simulink model "stereo_ibvs_core_before_04_kinematics_20260723_212009"  (R2025b)
settings: Solver=FixedStepDiscrete  StartTime=0.0  StopTime=inf  FixedStep=cfg.Ts  RelTol=1e-3
InitFcn:
  | cfgValid__=evalin('base','exist(''cfg'',''var'')==1 && isstruct(cfg) && all(isfield(cfg,{''Ts'',''robot'',''qInitial'',''zoomInitialSteps'',''cameraIntrinsicsStage1'',''rhoD'',''stereoBaseline'',''centerDesired'',''Kc'',''lambdaC'',''qMin'',''qMax'',''qLimitSoftMargin'',''qDotAlgorithmMax'',''stage1CalibrationReady''}))');if ~cfgValid__,modelFile__=get_param(bdroot,'FileName');modelDir__=fileparts(modelFile__);config1__=fullfile(modelDir__,'stereo_ibvs_config.m');config2__=fullfile(fileparts(modelDir__),'config','stereo_ibvs_config.m');if isfile(config1__),run(config1__);elseif isfile(config2__),run(config2__);else,error('StereoIBVS:ConfigNotFound','找不到stereo_ibvs_config.m。');end;end;clear cfgValid__ modelFile__ modelDir__ config1__ config2__
undefined symbols (not defined in the file): cfg
(part 1 of 2)
settings Model: Creator=harry  LastModifiedBy=harry

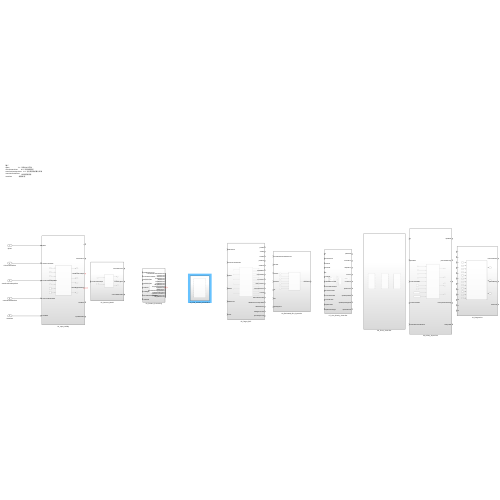
[thumbnail: Simulink's stored preview of the top-level diagram]
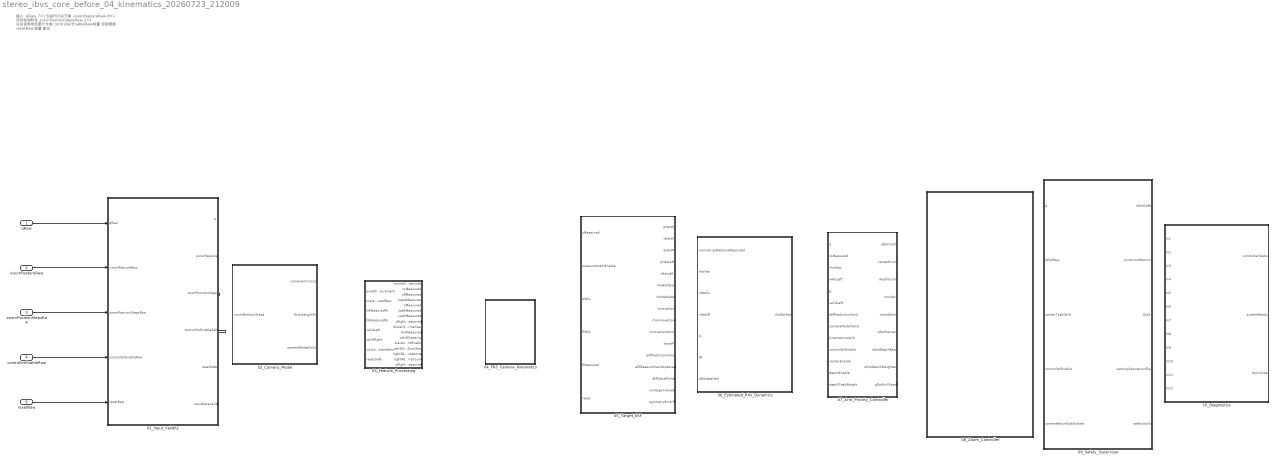
== system stereo_ibvs_core_before_04_kinematics_20260723_212009 ==
  note: 输入:
      | qRaw 7×1 当前FR3关节角
      | visionFeatureRaw 8×1 双目检测特征
      | zoomPositionStepsRaw 2×1 左右变焦电机累计步数
      | controllerEnableRaw 标量 控制使能
      | resetRaw 标量 复位
  qRaw : Inport  OutDataTypeStr=double  PortDimensions=[7 1]
  visionFeatureRaw : Inport  Port=2  PortDimensions=[8 1]
  zoomPositionStepsRaw : Inport  Port=3  PortDimensions=[2 1]
  controllerEnableRaw : Inport  Port=4  OutDataTypeStr=double  PortDimensions=1
  resetRaw : Inport  Port=5  OutDataTypeStr=double  PortDimensions=1
  01_Input_Validity : Subsystem
  02_Camera_Model : Subsystem
  03_Feature_Processing : Subsystem  Description=将像素坐标转换为左右相机归一化坐标，并检查输入有效性。
  04_FR3_Camera_Kinematics : Subsystem
  05_Target_EKF : Subsystem
  06_Estimated_Rho_Dynamics : Subsystem
  07_Arm_Priority_Controller : Subsystem
  08_Zoom_Controller : Subsystem
  09_Safety_Supervisor : Subsystem
  10_Diagnostics : Subsystem
  wires:
  resetRaw/1 -> 01_Input_Validity/5(resetRaw)
  controllerEnableRaw/1 -> 01_Input_Validity/4(controllerEnableRaw)
  zoomPositionStepsRaw/1 -> 01_Input_Validity/3(zoomPositionStepsRaw)
  visionFeatureRaw/1 -> 01_Input_Validity/2(visionFeatureRaw)
  01_Input_Validity/4(controllerEnableSafe) -> ?
  qRaw/1 -> 01_Input_Validity/1(qRaw)
  ? -> ?
  01_Input_Validity/3(zoomPositionSteps) -> ?

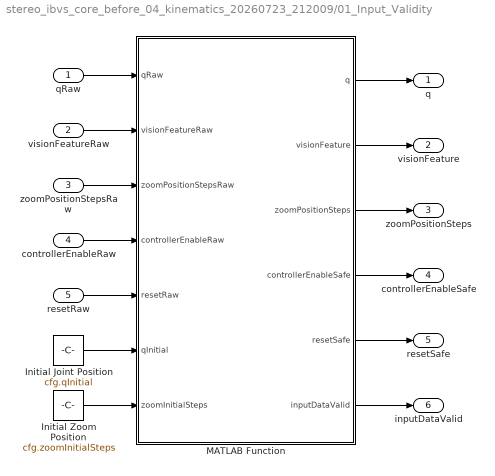
== system stereo_ibvs_core_before_04_kinematics_20260723_212009/01_Input_Validity ==
  qRaw : Inport  PortDimensions=[7 1]
  visionFeatureRaw : Inport  Port=2  PortDimensions=[8 1]
  zoomPositionStepsRaw : Inport  Port=3  PortDimensions=[2 1]
  controllerEnableRaw : Inport  Port=4  PortDimensions=1
  resetRaw : Inport  Port=5  PortDimensions=1
  Initial Joint Position : Constant  Value=cfg.qInitial  VectorParams1D=off
  Initial Zoom Position : Constant  Value=cfg.zoomInitialSteps  VectorParams1D=off
  MATLAB Function : MATLAB Function  TreatAsAtomicUnit=on
  q : Outport  PortDimensions=[7 1]
  visionFeature : Outport  Port=2  PortDimensions=[8 1]
  zoomPositionSteps : Outport  Port=3  PortDimensions=[2 1]
  controllerEnableSafe : Outport  Port=4  PortDimensions=1
  resetSafe : Outport  Port=5  PortDimensions=1
  inputDataValid : Outport  Port=6  PortDimensions=1
  wires:
  MATLAB Function/1(q) -> q/1
  MATLAB Function/2(visionFeature) -> visionFeature/1
  MATLAB Function/3(zoomPositionSteps) -> zoomPositionSteps/1
  MATLAB Function/4(controllerEnableSafe) -> controllerEnableSafe/1
  MATLAB Function/5(resetSafe) -> resetSafe/1
  MATLAB Function/6(inputDataValid) -> inputDataValid/1
  qRaw/1 -> MATLAB Function/1(qRaw)
  visionFeatureRaw/1 -> MATLAB Function/2(visionFeatureRaw)
  zoomPositionStepsRaw/1 -> MATLAB Function/3(zoomPositionStepsRaw)
  controllerEnableRaw/1 -> MATLAB Function/4(controllerEnableRaw)
  resetRaw/1 -> MATLAB Function/5(resetRaw)
  Initial Joint Position/1 -> MATLAB Function/6(qInitial)
  Initial Zoom Position/1 -> MATLAB Function/7(zoomInitialSteps)

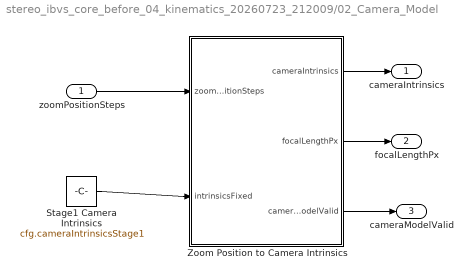
== system stereo_ibvs_core_before_04_kinematics_20260723_212009/02_Camera_Model ==
  zoomPositionSteps : Inport  PortDimensions=[2 1]
  Stage1 Camera Intrinsics : Constant  Value=cfg.cameraIntrinsicsStage1  VectorParams1D=off
  Zoom Position to Camera Intrinsics : MATLAB Function  TreatAsAtomicUnit=on
  cameraIntrinsics : Outport  PortDimensions=[8 1]
  focalLengthPx : Outport  Port=2  PortDimensions=[2 1]
  cameraModelValid : Outport  Port=3  PortDimensions=1
  wires:
  zoomPositionSteps/1 -> Zoom Position to Camera Intrinsics/1(zoomPositionSteps)
  Stage1 Camera Intrinsics/1 -> Zoom Position to Camera Intrinsics/2(intrinsicsFixed)
  Zoom Position to Camera Intrinsics/3(cameraModelValid) -> cameraModelValid/1
  Zoom Position to Camera Intrinsics/2(focalLengthPx) -> focalLengthPx/1
  Zoom Position to Camera Intrinsics/1(cameraIntrinsics) -> cameraIntrinsics/1

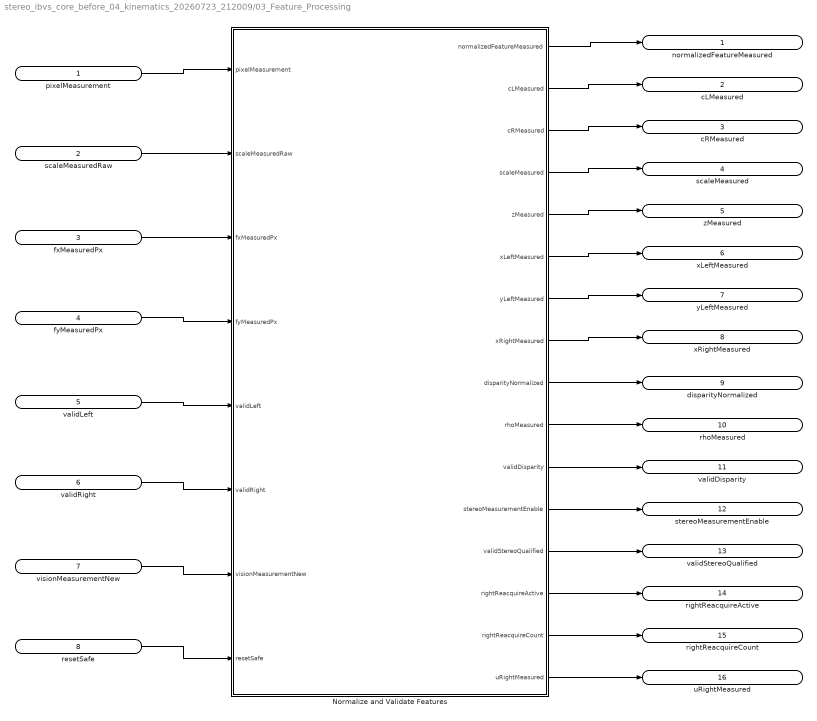
== system stereo_ibvs_core_before_04_kinematics_20260723_212009/03_Feature_Processing ==
  pixelMeasurement : Inport  OutDataTypeStr=double  PortDimensions=[4 1]
  scaleMeasuredRaw : Inport  Port=2  OutDataTypeStr=double  PortDimensions=[2 1]
  fxMeasuredPx : Inport  Port=3  OutDataTypeStr=double  PortDimensions=[2 1]
  fyMeasuredPx : Inport  Port=4  OutDataTypeStr=double  PortDimensions=[2 1]
  validLeft : Inport  Port=5  OutDataTypeStr=double  PortDimensions=[1 1]
  validRight : Inport  Port=6  OutDataTypeStr=double  PortDimensions=[1 1]
  visionMeasurementNew : Inport  Port=7  OutDataTypeStr=double  PortDimensions=[1 1]
  resetSafe : Inport  Port=8  OutDataTypeStr=double  PortDimensions=[1 1]
  Normalize and Validate Features : MATLAB Function  TreatAsAtomicUnit=on
  normalizedFeatureMeasured : Outport  PortDimensions=[4 1]
  cLMeasured : Outport  Port=2  PortDimensions=[2 1]
  cRMeasured : Outport  Port=3  PortDimensions=[2 1]
  scaleMeasured : Outport  Port=4  PortDimensions=[2 1]
  zMeasured : Outport  Port=5  PortDimensions=[3 1]
  xLeftMeasured : Outport  Port=6  PortDimensions=[1 1]
  yLeftMeasured : Outport  Port=7  PortDimensions=[1 1]
  xRightMeasured : Outport  Port=8  PortDimensions=[1 1]
  disparityNormalized : Outport  Port=9  PortDimensions=[1 1]
  rhoMeasured : Outport  Port=10  PortDimensions=[1 1]
  validDisparity : Outport  Port=11  PortDimensions=[1 1]
  stereoMeasurementEnable : Outport  Port=12  PortDimensions=[1 1]
  validStereoQualified : Outport  Port=13  PortDimensions=[1 1]
  rightReacquireActive : Outport  Port=14  PortDimensions=[1 1]
  rightReacquireCount : Outport  Port=15  PortDimensions=[1 1]
  uRightMeasured : Outport  Port=16  PortDimensions=[1 1]
  wires:
  pixelMeasurement/1 -> Normalize and Validate Features/1(pixelMeasurement)
  scaleMeasuredRaw/1 -> Normalize and Validate Features/2(scaleMeasuredRaw)
  fxMeasuredPx/1 -> Normalize and Validate Features/3(fxMeasuredPx)
  fyMeasuredPx/1 -> Normalize and Validate Features/4(fyMeasuredPx)
  validLeft/1 -> Normalize and Validate Features/5(validLeft)
  validRight/1 -> Normalize and Validate Features/6(validRight)
  visionMeasurementNew/1 -> Normalize and Validate Features/7(visionMeasurementNew)
  resetSafe/1 -> Normalize and Validate Features/8(resetSafe)
  Normalize and Validate Features/2(cLMeasured) -> cLMeasured/1
  Normalize and Validate Features/3(cRMeasured) -> cRMeasured/1
  Normalize and Validate Features/4(scaleMeasured) -> scaleMeasured/1
  Normalize and Validate Features/5(zMeasured) -> zMeasured/1
  Normalize and Validate Features/6(xLeftMeasured) -> xLeftMeasured/1
  Normalize and Validate Features/7(yLeftMeasured) -> yLeftMeasured/1
  Normalize and Validate Features/8(xRightMeasured) -> xRightMeasured/1
  Normalize and Validate Features/9(disparityNormalized) -> disparityNormalized/1
  Normalize and Validate Features/10(rhoMeasured) -> rhoMeasured/1
  Normalize and Validate Features/11(validDisparity) -> validDisparity/1
  Normalize and Validate Features/12(stereoMeasurementEnable) -> stereoMeasurementEnable/1
  Normalize and Validate Features/13(validStereoQualified) -> validStereoQualified/1
  Normalize and Validate Features/14(rightReacquireActive) -> rightReacquireActive/1
  Normalize and Validate Features/15(rightReacquireCount) -> rightReacquireCount/1
  Normalize and Validate Features/16(uRightMeasured) -> uRightMeasured/1
  Normalize and Validate Features/1(normalizedFeatureMeasured) -> normalizedFeatureMeasured/1

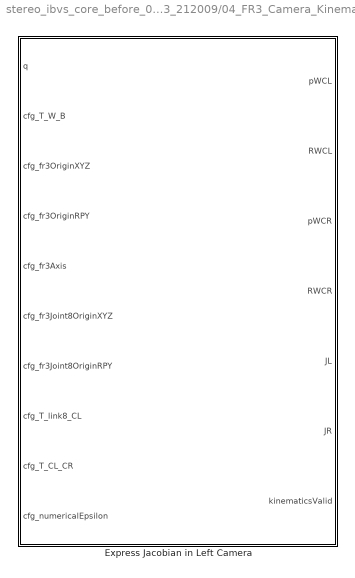
== system stereo_ibvs_core_before_04_kinematics_20260723_212009/04_FR3_Camera_Kinematics ==
  Express Jacobian in Left Camera : MATLAB Function  TreatAsAtomicUnit=on

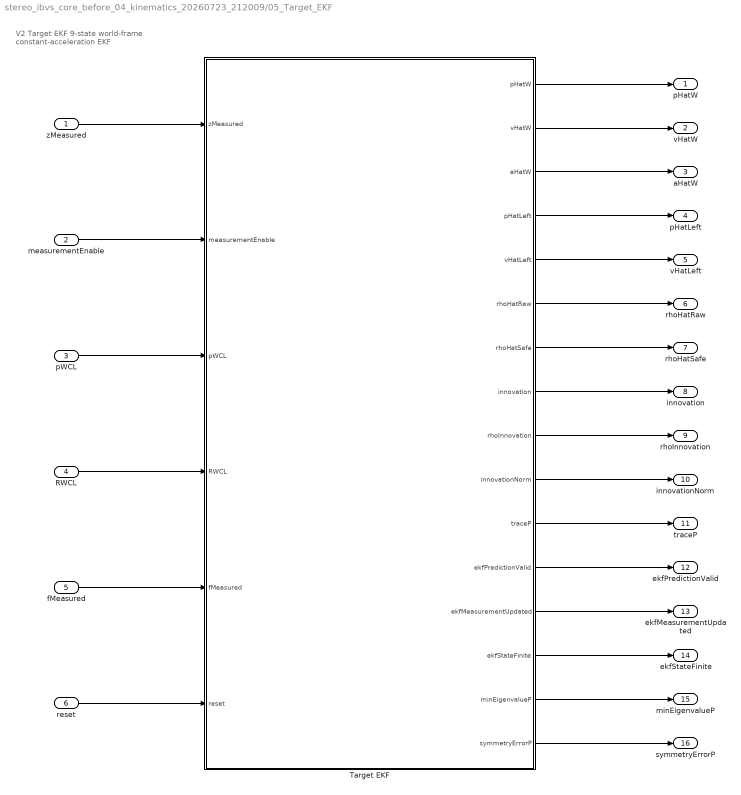
== system stereo_ibvs_core_before_04_kinematics_20260723_212009/05_Target_EKF ==
  note: V2 Target EKF
      | 9-state world-frame constant-acceleration EKF
  zMeasured : Inport  OutDataTypeStr=double  PortDimensions=3
  measurementEnable : Inport  Port=2  OutDataTypeStr=double  PortDimensions=1
  pWCL : Inport  Port=3  OutDataTypeStr=double  PortDimensions=3
  RWCL : Inport  Port=4  OutDataTypeStr=double  PortDimensions=[3 3]
  fMeasured : Inport  Port=5  OutDataTypeStr=double  PortDimensions=2
  reset : Inport  Port=6  OutDataTypeStr=double  PortDimensions=1
  Target EKF : MATLAB Function  TreatAsAtomicUnit=on
  pHatW : Outport
  vHatW : Outport  Port=2
  aHatW : Outport  Port=3
  pHatLeft : Outport  Port=4
  vHatLeft : Outport  Port=5
  rhoHatRaw : Outport  Port=6
  rhoHatSafe : Outport  Port=7
  innovation : Outport  Port=8
  rhoInnovation : Outport  Port=9
  innovationNorm : Outport  Port=10
  traceP : Outport  Port=11
  ekfPredictionValid : Outport  Port=12
  ekfMeasurementUpdated : Outport  Port=13
  ekfStateFinite : Outport  Port=14
  minEigenvalueP : Outport  Port=15
  symmetryErrorP : Outport  Port=16
  wires:
  zMeasured/1 -> Target EKF/1(zMeasured)
  measurementEnable/1 -> Target EKF/2(measurementEnable)
  pWCL/1 -> Target EKF/3(pWCL)
  RWCL/1 -> Target EKF/4(RWCL)
  fMeasured/1 -> Target EKF/5(fMeasured)
  reset/1 -> Target EKF/6(reset)
  Target EKF/1(pHatW) -> pHatW/1
  Target EKF/2(vHatW) -> vHatW/1
  Target EKF/3(aHatW) -> aHatW/1
  Target EKF/4(pHatLeft) -> pHatLeft/1
  Target EKF/5(vHatLeft) -> vHatLeft/1
  Target EKF/6(rhoHatRaw) -> rhoHatRaw/1
  Target EKF/7(rhoHatSafe) -> rhoHatSafe/1
  Target EKF/8(innovation) -> innovation/1
  Target EKF/9(rhoInnovation) -> rhoInnovation/1
  Target EKF/10(innovationNorm) -> innovationNorm/1
  Target EKF/11(traceP) -> traceP/1
  Target EKF/12(ekfPredictionValid) -> ekfPredictionValid/1
  Target EKF/13(ekfMeasurementUpdated) -> ekfMeasurementUpdated/1
  Target EKF/14(ekfStateFinite) -> ekfStateFinite/1
  Target EKF/15(minEigenvalueP) -> minEigenvalueP/1
  Target EKF/16(symmetryErrorP) -> symmetryErrorP/1

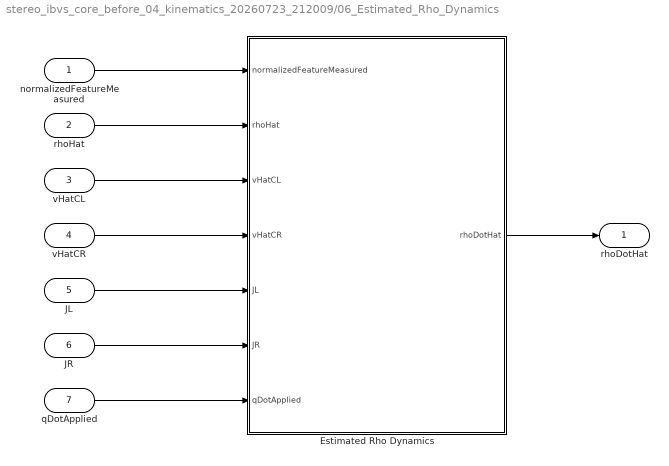
== system stereo_ibvs_core_before_04_kinematics_20260723_212009/06_Estimated_Rho_Dynamics ==
  normalizedFeatureMeasured : Inport  OutDataTypeStr=double  PortDimensions=[4 1]
  rhoHat : Inport  Port=2  OutDataTypeStr=double  PortDimensions=1
  vHatCL : Inport  Port=3  OutDataTypeStr=double  PortDimensions=[3 1]
  vHatCR : Inport  Port=4  OutDataTypeStr=double  PortDimensions=[3 1]
  JL : Inport  Port=5  OutDataTypeStr=double  PortDimensions=[6 7]
  JR : Inport  Port=6  OutDataTypeStr=double  PortDimensions=[6 7]
  qDotApplied : Inport  Port=7  OutDataTypeStr=double  PortDimensions=[7 1]
  Estimated Rho Dynamics : MATLAB Function  TreatAsAtomicUnit=on
  rhoDotHat : Outport  OutDataTypeStr=double  PortDimensions=[2 1]
  wires:
  normalizedFeatureMeasured/1 -> Estimated Rho Dynamics/1(normalizedFeatureMeasured)
  rhoHat/1 -> Estimated Rho Dynamics/2(rhoHat)
  vHatCL/1 -> Estimated Rho Dynamics/3(vHatCL)
  vHatCR/1 -> Estimated Rho Dynamics/4(vHatCR)
  JL/1 -> Estimated Rho Dynamics/5(JL)
  JR/1 -> Estimated Rho Dynamics/6(JR)
  qDotApplied/1 -> Estimated Rho Dynamics/7(qDotApplied)
  Estimated Rho Dynamics/1(rhoDotHat) -> rhoDotHat/1

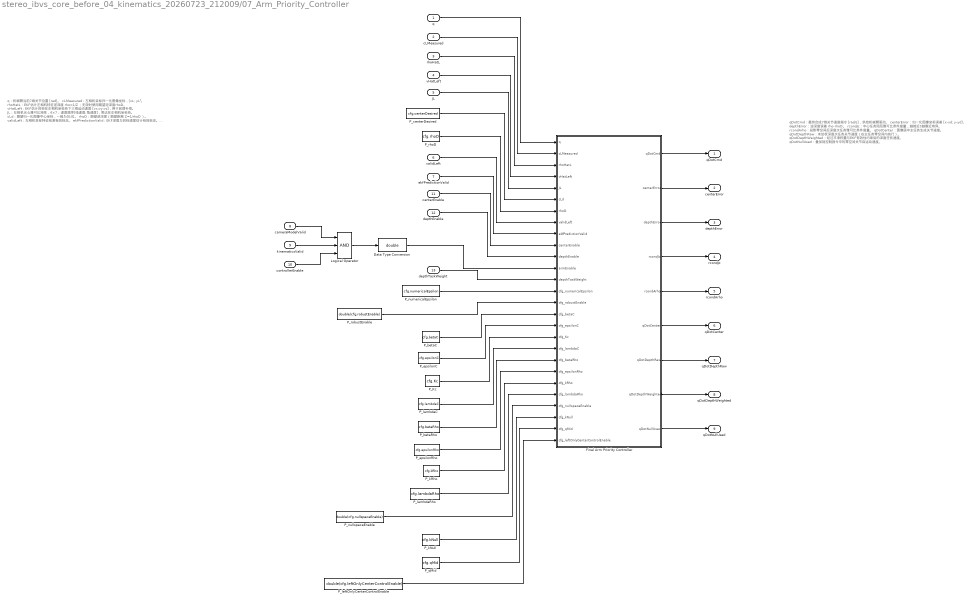
== system stereo_ibvs_core_before_04_kinematics_20260723_212009/07_Arm_Priority_Controller ==
  note: qDotCmd：最终合成7维关节速度指令 [rad/s]，供给机械臂驱动。
      | centerError：归一化图像坐标误差 [x-xd; y-yd]。
      | depthError：逆深度误差 rho-rhoD。
      | rcondJc：中心任务阻尼雅可比条件度量，越接近0越靠近奇异。
      | rcondArho：投影零空间后深度次任务雅可比条件度量。
      | qDotCenter：图像居中主任务生成关节速度。
      | qDotDepthRaw：未加权深度次任务关节速度（在主任务零空间内执行）。
      | qDotDepthWeighted：经过平滑权重与EKF有效性约束后的深度任务速度。
      | qDotNullUsed：叠加到控制指令中的零空间关节自运动速度。
  note: q：机械臂当前7维关节位置 [rad]。
      | cLMeasured：左相机目标归一化图像坐标，[xL; yL]。
      | rhoHatL：EKF估计左相机特征逆深度 rho=1/Z；无效时使用期望逆深度rhoD。
      | vHatLeft：EKF估计目标在左相机坐标系下三维运动速度 [vx;vy;vz]，用于前馈补偿。
      | JL：左相机光心雅可比矩阵，6×7；速度顺序[线速度;角速度]，表达在左相机坐标系。
      | cLd：期望归一化图像中心坐标，一般为[0;0]。
      | rhoD：期望逆深度（期望距离 Z=1/rhoD）。
      | validLeft：左相机目标特征检测有效标志。
      | ekfPredictionValid：EKF深度与目标速度估计有效标志。
      | centerEnable：图像居中主任务使能。
      | depthEnable：逆深度（距离调节）次任务使能。
      | armEnable：机械臂控制器总使能开关。
      | depthTaskWeight：深度次任务平滑权重，范围[0,1]，用于任务软切换抑制冲击。
      | cfg_numericalEpsilon：数值计算最小阈值，防止除零奇异。
      | cfg_robustEnable：鲁棒误差项开关；开启后限制大误差下指令激增。
      | cfg_betaC：中心任务鲁棒核系数。
      | cfg_epsilonC：中心任务鲁棒核正则小量。
      | cfg_Kc：图像居中主任务反馈增益。
      | cfg_lambdaC：中心任务阻尼伪逆系数。
      | cfg_betaRho：深度任务鲁棒核系数。
      | cfg_epsilonRho：深度任务鲁棒核正则小量。
      | cfg_kRho：逆深度距离调节反馈增益。
      | cfg_lambdaRho：深度次任务阻尼伪逆系数。
      | cfg_nullspaceEnable：零空间关节自运动任务使能。
      | cfg_kNull：零空间关节中位回归增益。
      | cfg_qMid：机械臂关节中位参考位置，用于零空间自运动。
      | cfg_leftOnlyCenterControlEnable：仅允许左相机视觉控制标志。
  q : Inport  PortDimensions=[7 1]
  cLMeasured : Inport  Port=2  PortDimensions=[2 1]
  rhoHatL : Inport  Port=3  PortDimensions=1
  vHatLeft : Inport  Port=4  PortDimensions=[3 1]
  JL : Inport  Port=5  PortDimensions=[6 7]
  validLeft : Inport  Port=6  PortDimensions=1
  ekfPredictionValid : Inport  Port=7  PortDimensions=1
  cameraModelValid : Inport  Port=8  PortDimensions=1
  kinematicsValid : Inport  Port=9  PortDimensions=1
  controllerEnable : Inport  Port=10  PortDimensions=1
  centerEnable : Inport  Port=11  PortDimensions=1
  depthEnable : Inport  Port=12  PortDimensions=1
  depthTaskWeight : Inport  Port=13  PortDimensions=1
  Data Type Conversion : DataTypeConversion  OutDataTypeStr=double  SaturateOnIntegerOverflow=off  RndMeth=Floor
  Final Arm Priority Controller : MATLAB Function  TreatAsAtomicUnit=on
  Logical Operator : Logic  Inputs=3  AllPortsSameDT=off  OutDataTypeStr=boolean
  P_Kc : Constant  Value=cfg.Kc  VectorParams1D=off  SampleTime=-1
  P_betaC : Constant  Value=cfg.betaC  VectorParams1D=off  SampleTime=-1
  P_betaRho : Constant  Value=cfg.betaRho  VectorParams1D=off  SampleTime=-1
  P_centerDesired : Constant  Value=cfg.centerDesired  VectorParams1D=off  SampleTime=-1
  P_epsilonC : Constant  Value=cfg.epsilonC  VectorParams1D=off  SampleTime=-1
  P_epsilonRho : Constant  Value=cfg.epsilonRho  VectorParams1D=off  SampleTime=-1
  P_kNull : Constant  Value=cfg.kNull  VectorParams1D=off  SampleTime=-1
  P_kRho : Constant  Value=cfg.kRho  VectorParams1D=off  SampleTime=-1
  P_lambdaC : Constant  Value=cfg.lambdaC  VectorParams1D=off  SampleTime=-1
  P_lambdaRho : Constant  Value=cfg.lambdaRho  VectorParams1D=off  SampleTime=-1
  P_leftOnlyCenterControlEnable : Constant  Value=double(cfg.leftOnlyCenterControlEnable)  VectorParams1D=off  SampleTime=-1
  P_nullspaceEnable : Constant  Value=double(cfg.nullspaceEnable)  VectorParams1D=off  SampleTime=-1
  P_numericalEpsilon : Constant  Value=cfg.numericalEpsilon  VectorParams1D=off  SampleTime=-1
  P_qMid : Constant  Value=cfg.qMid  VectorParams1D=off  SampleTime=-1
  P_rhoD : Constant  Value=cfg.rhoD  VectorParams1D=off  SampleTime=-1
  P_robustEnable : Constant  Value=double(cfg.robustEnable)  VectorParams1D=off  SampleTime=-1
  qDotCmd : Outport  PortDimensions=[7 1]
  centerError : Outport  Port=2  PortDimensions=[2 1]
  depthError : Outport  Port=3  PortDimensions=1
  rcondJc : Outport  Port=4  PortDimensions=1
  rcondArho : Outport  Port=5  PortDimensions=1
  qDotCenter : Outport  Port=6  PortDimensions=[7 1]
  qDotDepthRaw : Outport  Port=7  PortDimensions=[7 1]
  qDotDepthWeighted : Outport  Port=8  PortDimensions=[7 1]
  qDotNullUsed : Outport  Port=9  PortDimensions=[7 1]
  wires:
  Final Arm Priority Controller/8(qDotDepthWeighted) -> qDotDepthWeighted/1
  Final Arm Priority Controller/7(qDotDepthRaw) -> qDotDepthRaw/1
  Final Arm Priority Controller/5(rcondArho) -> rcondArho/1
  Final Arm Priority Controller/3(depthError) -> depthError/1
  Final Arm Priority Controller/2(centerError) -> centerError/1
  Final Arm Priority Controller/1(qDotCmd) -> qDotCmd/1
  validLeft/1 -> Final Arm Priority Controller/8(validLeft)
  P_rhoD/1 -> Final Arm Priority Controller/7(rhoD)
  P_betaC/1 -> Final Arm Priority Controller/16(cfg_betaC)
  P_centerDesired/1 -> Final Arm Priority Controller/6(cLd)
  P_leftOnlyCenterControlEnable/1 -> Final Arm Priority Controller/27(cfg_leftOnlyCenterControlEnable)
  P_kRho/1 -> Final Arm Priority Controller/22(cfg_kRho)
  Final Arm Priority Controller/4(rcondJc) -> rcondJc/1
  JL/1 -> Final Arm Priority Controller/5(JL)
  ekfPredictionValid/1 -> Final Arm Priority Controller/9(ekfPredictionValid)
  P_lambdaC/1 -> Final Arm Priority Controller/19(cfg_lambdaC)
  vHatLeft/1 -> Final Arm Priority Controller/4(vHatLeft)
  depthEnable/1 -> Final Arm Priority Controller/11(depthEnable)
  cLMeasured/1 -> Final Arm Priority Controller/2(cLMeasured)
  q/1 -> Final Arm Priority Controller/1(q)
  controllerEnable/1 -> Logical Operator/3
  P_betaRho/1 -> Final Arm Priority Controller/20(cfg_betaRho)
  Final Arm Priority Controller/6(qDotCenter) -> qDotCenter/1
  centerEnable/1 -> Final Arm Priority Controller/10(centerEnable)
  P_epsilonC/1 -> Final Arm Priority Controller/17(cfg_epsilonC)
  kinematicsValid/1 -> Logical Operator/2
  cameraModelValid/1 -> Logical Operator/1
  rhoHatL/1 -> Final Arm Priority Controller/3(rhoHatL)
  depthTaskWeight/1 -> Final Arm Priority Controller/13(depthTaskWeight)
  P_numericalEpsilon/1 -> Final Arm Priority Controller/14(cfg_numericalEpsilon)
  P_Kc/1 -> Final Arm Priority Controller/18(cfg_Kc)
  P_epsilonRho/1 -> Final Arm Priority Controller/21(cfg_epsilonRho)
  P_robustEnable/1 -> Final Arm Priority Controller/15(cfg_robustEnable)
  P_lambdaRho/1 -> Final Arm Priority Controller/23(cfg_lambdaRho)
  P_nullspaceEnable/1 -> Final Arm Priority Controller/24(cfg_nullspaceEnable)
  P_kNull/1 -> Final Arm Priority Controller/25(cfg_kNull)
  Final Arm Priority Controller/9(qDotNullUsed) -> qDotNullUsed/1
  P_qMid/1 -> Final Arm Priority Controller/26(cfg_qMid)
  Logical Operator/1 -> Data Type Conversion/1
  Data Type Conversion/1 -> Final Arm Priority Controller/12(armEnable)

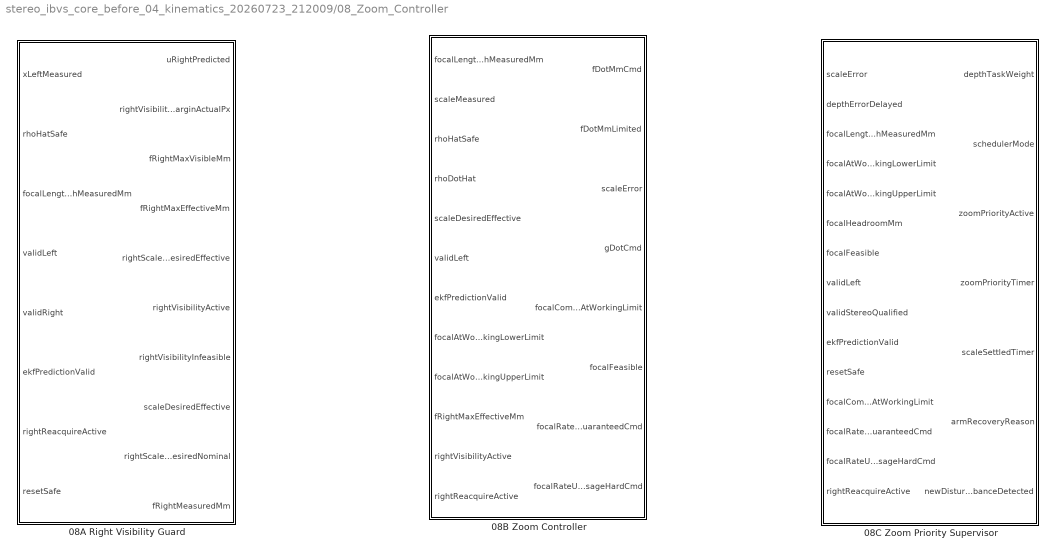
== system stereo_ibvs_core_before_04_kinematics_20260723_212009/08_Zoom_Controller ==
  08A Right Visibility Guard : MATLAB Function  TreatAsAtomicUnit=on
  08B Zoom Controller : MATLAB Function  TreatAsAtomicUnit=on
  08C Zoom Priority Supervisor : MATLAB Function  TreatAsAtomicUnit=on

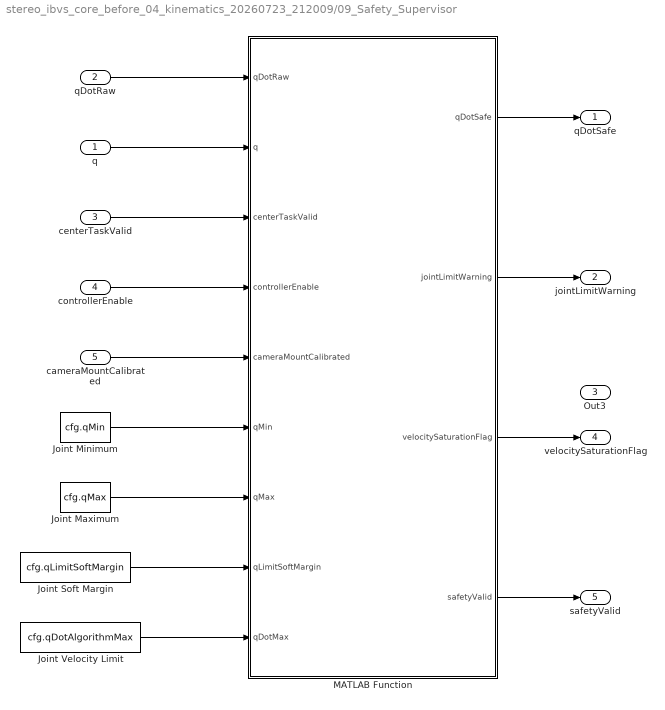
== system stereo_ibvs_core_before_04_kinematics_20260723_212009/09_Safety_Supervisor ==
  q : Inport  PortDimensions=[7 1]
  qDotRaw : Inport  Port=2  PortDimensions=[7 1]
  centerTaskValid : Inport  Port=3  PortDimensions=1
  controllerEnable : Inport  Port=4  PortDimensions=1
  cameraMountCalibrated : Inport  Port=5  PortDimensions=1
  Joint Maximum : Constant  Value=cfg.qMax  VectorParams1D=off
  Joint Minimum : Constant  Value=cfg.qMin  VectorParams1D=off
  Joint Soft Margin : Constant  Value=cfg.qLimitSoftMargin  VectorParams1D=off
  Joint Velocity Limit : Constant  Value=cfg.qDotAlgorithmMax  VectorParams1D=off
  MATLAB Function : MATLAB Function  TreatAsAtomicUnit=on
  qDotSafe : Outport  PortDimensions=[7 1]
  jointLimitWarning : Outport  Port=2  PortDimensions=[7 1]
  Out3 : Outport  Port=3
  velocitySaturationFlag : Outport  Port=4  PortDimensions=[7 1]
  safetyValid : Outport  Port=5  PortDimensions=1
  wires:
  MATLAB Function/2(jointLimitWarning) -> jointLimitWarning/1
  MATLAB Function/3(velocitySaturationFlag) -> velocitySaturationFlag/1
  MATLAB Function/1(qDotSafe) -> qDotSafe/1
  Joint Velocity Limit/1 -> MATLAB Function/9(qDotMax)
  MATLAB Function/4(safetyValid) -> safetyValid/1
  Joint Maximum/1 -> MATLAB Function/7(qMax)
  Joint Minimum/1 -> MATLAB Function/6(qMin)
  controllerEnable/1 -> MATLAB Function/4(controllerEnable)
  Joint Soft Margin/1 -> MATLAB Function/8(qLimitSoftMargin)
  centerTaskValid/1 -> MATLAB Function/3(centerTaskValid)
  cameraMountCalibrated/1 -> MATLAB Function/5(cameraMountCalibrated)
  q/1 -> MATLAB Function/2(q)
  qDotRaw/1 -> MATLAB Function/1(qDotRaw)

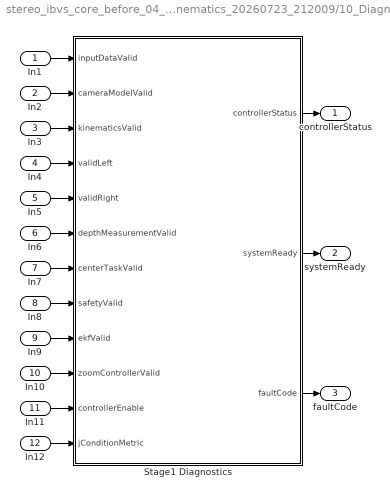
== system stereo_ibvs_core_before_04_kinematics_20260723_212009/10_Diagnostics ==
  In1 : Inport  PortDimensions=1
  In2 : Inport  Port=2  PortDimensions=1
  In3 : Inport  Port=3  PortDimensions=1
  In4 : Inport  Port=4  PortDimensions=1
  In5 : Inport  Port=5  PortDimensions=1
  In6 : Inport  Port=6  PortDimensions=1
  In7 : Inport  Port=7  PortDimensions=1
  In8 : Inport  Port=8  PortDimensions=1
  In9 : Inport  Port=9  PortDimensions=1
  In10 : Inport  Port=10  PortDimensions=1
  In11 : Inport  Port=11  PortDimensions=1
  In12 : Inport  Port=12  PortDimensions=1
  Stage1 Diagnostics : MATLAB Function  TreatAsAtomicUnit=on
  controllerStatus : Outport  PortDimensions=[12 1]
  systemReady : Outport  Port=2  PortDimensions=1
  faultCode : Outport  Port=3  PortDimensions=1
  wires:
  In1/1 -> Stage1 Diagnostics/1(inputDataValid)
  In2/1 -> Stage1 Diagnostics/2(cameraModelValid)
  In3/1 -> Stage1 Diagnostics/3(kinematicsValid)
  In4/1 -> Stage1 Diagnostics/4(validLeft)
  In5/1 -> Stage1 Diagnostics/5(validRight)
  In6/1 -> Stage1 Diagnostics/6(depthMeasurementValid)
  In7/1 -> Stage1 Diagnostics/7(centerTaskValid)
  In8/1 -> Stage1 Diagnostics/8(safetyValid)
  In9/1 -> Stage1 Diagnostics/9(ekfValid)
  In10/1 -> Stage1 Diagnostics/10(zoomControllerValid)
  In11/1 -> Stage1 Diagnostics/11(controllerEnable)
  In12/1 -> Stage1 Diagnostics/12(jConditionMetric)
  Stage1 Diagnostics/1(controllerStatus) -> controllerStatus/1
  Stage1 Diagnostics/2(systemReady) -> systemReady/1
  Stage1 Diagnostics/3(faultCode) -> faultCode/1

== matlab function stereo_ibvs_core_before_04_kinematics_20260723_212009/09_Safety_Supervisor/MATLAB Function ==
  data: qDotRaw input; qDotSafe output; q input; centerTaskValid input; controllerEnable input; cameraMountCalibrated input; qMin input; qMax input; qLimitSoftMargin input; qDotMax input; jointLimitWarning output; velocitySaturationFlag output; safetyValid output
function [qDotSafe,jointLimitWarning,velocitySaturationFlag,safetyValid] = ...
    fcn(qDotRaw,q,centerTaskValid,controllerEnable,cameraMountCalibrated, ...
    qMin,qMax,qLimitSoftMargin,qDotMax)
%#codegen
% 代码作用：
% 对控制器产生的7维关节速度进行有限值检查、速度限幅和关节软限位保护。
% 当输入无效、控制器未使能或手眼标定未完成时，输出零关节速度。

% 输入参数含义：
% qDotRaw：
% 控制器计算出的原始7维关节速度，单位rad/s。
%
% q：
% 当前FR3的7维关节位置，单位rad。
%
% centerTaskValid：
% 中心任务本次计算是否有效。
%
% controllerEnable：
% 控制器总使能信号。
%
% cameraMountCalibrated：
% 左相机与fr3_link8之间的手眼安装矩阵是否已经完成标定。
%
% qMin、qMax：
% FR3七个关节的最小和最大允许位置，单位rad。
%
% qLimitSoftMargin：
% 关节软限位保护距离，单位rad。
%
% qDotMax：
% Simulink算法层允许的最大关节速度，单位rad/s。

% 输出参数含义：
% qDotSafe：
% 经过安全检查后的7维关节速度，单位rad/s。
%
% jointLimitWarning：
% 每个关节是否进入软限位区域，进入为1，否则为0。
%
% velocitySaturationFlag：
% 每个关节是否发生速度限幅，发生为1，否则为0。
%
% safetyValid：
% 当前是否允许输出非零关节速度，允许为1，否则为0。

qDotSafe = zeros(7,1);
jointLimitWarning = zeros(7,1);
velocitySaturationFlag = zeros(7,1);
safetyValid = 0;

qDotCandidate = reshape(qDotRaw,7,1);
qCurrent = reshape(q,7,1);
qLower = reshape(qMin,7,1);
qUpper = reshape(qMax,7,1);
qDotLimit = reshape(qDotMax,7,1);

% 检查输入是否包含NaN或Inf。
if any(~isfinite(qDotCandidate)) || ...
        any(~isfinite(qCurrent)) || ...
        any(~isfinite(qLower)) || ...
        any(~isfinite(qUpper)) || ...
        any(~isfinite(qDotLimit)) || ...
        ~isfinite(qLimitSoftMargin)
    return;
end

% 检查控制链路是否允许输出速度。
if centerTaskValid <= 0.5 || ...
        controllerEnable <= 0.5 || ...
        cameraMountCalibrated <= 0.5
    return;
end

if qLimitSoftMargin <= 0 || ...
        any(qUpper <= qLower) || ...
        any(qDotLimit <= 0)
    return;
end

% 关节速度逐元素限幅。
qDotLimited = min(max(qDotCandidate,-qDotLimit),qDotLimit);

velocitySaturationFlag = double( ...
    abs(qDotLimited-qDotCandidate) > 1e-12);

% 关节软限位保护。
for i = 1:7
    nearLowerLimit = ...
        qCurrent(i)-qLower(i) <= qLimitSoftMargin;

    nearUpperLimit = ...
        qUpper(i)-qCurrent(i) <= qLimitSoftMargin;

    jointLimitWarning(i) = double( ...
        nearLowerLimit || nearUpperLimit);

    % 接近下限时，禁止继续向下限方向运动。
    if nearLowerLimit && qDotLimited(i) < 0
        qDotLimited(i) = 0;
    end

    % 接近上限时，禁止继续向上限方向运动。
    if nearUpperLimit && qDotLimited(i) > 0
        qDotLimited(i) = 0;
    end

    % 已经越过硬限位时，同样禁止继续向外运动。
    if qCurrent(i) <= qLower(i) && qDotLimited(i) < 0
        qDotLimited(i) = 0;
    end

    if qCurrent(i) >= qUpper(i) && qDotLimited(i) > 0
        qDotLimited(i) = 0;
    end
end

if any(~isfinite(qDotLimited))
    return;
end

qDotSafe = qDotLimited;
safetyValid = 1;
end

== matlab function stereo_ibvs_core_before_04_kinematics_20260723_212009/01_Input_Validity/MATLAB Function ==
  data: qRaw input; q output; visionFeatureRaw input; zoomPositionStepsRaw input; controllerEnableRaw input; resetRaw input; qInitial input; zoomInitialSteps input; visionFeature output; zoomPositionSteps output; controllerEnableSafe output; resetSafe output; inputDataValid output
function [q,visionFeature,zoomPositionSteps,controllerEnableSafe, ...
    resetSafe,inputDataValid] = ...
    fcn(qRaw,visionFeatureRaw,zoomPositionStepsRaw, ...
    controllerEnableRaw,resetRaw,qInitial,zoomInitialSteps)
%#codegen
% 代码作用：
% 检查模型顶层输入是否包含NaN或Inf。
% 合法输入会被保存；非法输入使用最近一次合法值代替，
% 同时关闭控制器，防止无效数据进入运动学和控制模块。

% 输入参数含义：
% qRaw：
% ROS或仿真输入的FR3七维关节位置，单位rad。
%
% visionFeatureRaw：
% 双目视觉特征，格式为：
% [validL; validR; uL; vL; uR; vR; scaleL; scaleR]
%
% zoomPositionStepsRaw：
% 左右变焦步进电机累计位置：
% [leftSteps; rightSteps]
%
% controllerEnableRaw：
% 外部控制器使能信号。
%
% resetRaw：
% 控制器和估计器复位信号。
%
% qInitial：
% 输入无效时使用的初始安全关节位置。
%
% zoomInitialSteps：
% 输入无效时使用的初始变焦电机位置。

% 输出参数含义：
% q：
% 检查后的七维关节位置。
%
% visionFeature：
% 检查后的双目视觉特征。
%
% zoomPositionSteps：
% 检查后的左右变焦电机累计位置。
%
% controllerEnableSafe：
% 安全控制使能。只有全部输入有效时才允许为1。
%
% resetSafe：
% 检查后的复位信号。
%
% inputDataValid：
% 本周期全部输入是否有效，有效为1，无效为0。

persistent lastQ
persistent lastVisionFeature
persistent lastZoomPositionSteps

initialQ = reshape(qInitial,7,1);
initialZoom = reshape(zoomInitialSteps,2,1);

if isempty(lastQ)
    lastQ = initialQ;
    lastVisionFeature = zeros(8,1);
    lastZoomPositionSteps = initialZoom;
end

qCandidate = reshape(qRaw,7,1);
visionCandidate = reshape(visionFeatureRaw,8,1);
zoomCandidate = reshape(zoomPositionStepsRaw,2,1);

qValid = all(isfinite(qCandidate));
visionValid = all(isfinite(visionCandidate));
zoomValid = all(isfinite(zoomCandidate));
enableValid = isfinite(controllerEnableRaw);
resetValid = isfinite(resetRaw);

if qValid
    lastQ = qCandidate;
end

if visionValid
    lastVisionFeature = visionCandidate;
end

if zoomValid
    lastZoomPositionSteps = zoomCandidate;
end

q = lastQ;
visionFeature = lastVisionFeature;
zoomPositionSteps = lastZoomPositionSteps;

inputDataValid = double( ...
    qValid && ...
    visionValid && ...
    zoomValid && ...
    enableValid && ...
    resetValid);

controllerEnableSafe = double( ...
    inputDataValid > 0.5 && ...
    controllerEnableRaw > 0.5);

if resetValid
    resetSafe = double(resetRaw > 0.5);
else
    resetSafe = 0;
end

% 复位时清除历史输入。
if resetSafe > 0.5
    lastQ = initialQ;
    lastVisionFeature = zeros(8,1);
    lastZoomPositionSteps = initialZoom;

    q = lastQ;
    visionFeature = lastVisionFeature;
    zoomPositionSteps = lastZoomPositionSteps;
    controllerEnableSafe = 0;
end
end

== matlab function stereo_ibvs_core_before_04_kinematics_20260723_212009/06_Estimated_Rho_Dynamics/Estimated Rho Dynamics ==
  data: normalizedFeatureMeasured input double size=[4 1]; rhoDotHat output double size=[2 1]; rhoHat input double size=1; vHatCL input double size=[3 1]; vHatCR input double size=[3 1]; JL input double size=[6 7]; JR input double size=[6 7]; qDotApplied input double size=[7 1]
function rhoDotHat = fcn( ...
    normalizedFeatureMeasured, ...
    rhoHat, ...
    vHatCL, ...
    vHatCR, ...
    JL, ...
    JR, ...
    qDotApplied)
%#codegen
% V2逆深度变化率预测。
%
% normalizedFeatureMeasured:
% [xLeft; yLeft; xRight; yRight]
%
% rhoHat：
% EKF输出的安全逆深度。
%
% rhoDotHat：
% [rhoDotHatLeft; rhoDotHatRight]

%% 固定尺寸输出
rhoDotHat = zeros(2,1);

%% 左右相机逆深度动态
for cameraIndex = 1:2

    if cameraIndex == 1
        x = normalizedFeatureMeasured(1);
        y = normalizedFeatureMeasured(2);

        rho = max( ...
            rhoHat, ...
            cfg_numericalEpsilon);

        J = JL;
        targetVelocity = vHatCL;

    else
        x = normalizedFeatureMeasured(3);
        y = normalizedFeatureMeasured(4);

        rho = max( ...
            rhoHat, ...
            cfg_numericalEpsilon);

        J = JR;
        targetVelocity = vHatCR;
    end

    % 相机运动对逆深度的影响。
    Lrho = [
        0, ...
        0, ...
        rho*rho, ...
        rho*y, ...
        -rho*x, ...
        0
    ];

    % 目标平移速度对逆深度的影响。
    Hrho = [
        0, ...
        0, ...
        -rho*rho
    ];

    cameraVelocity = J * qDotApplied;

    rhoDotHat(cameraIndex) = ...
        Lrho * cameraVelocity + ...
        Hrho * targetVelocity;
end

%% 数值保护
if any(~isfinite(rhoDotHat))
    rhoDotHat = zeros(2,1);
end
end

== matlab function stereo_ibvs_core_before_04_kinematics_20260723_212009/05_Target_EKF/Target EKF ==
  data: zMeasured input double size=[3 1]; pHatW output double size=[3 1]; measurementEnable input double size=1; pWCL input double size=[3 1]; RWCL input double size=[3 3]; fMeasured input double size=[2 1]; reset input double size=1; vHatW output double size=[3 1]; aHatW output double size=[3 1]; pHatLeft output double size=[3 1]; vHatLeft output double size=[3 1]; rhoHatRaw output double size=1; rhoHatSafe output double size=1; innovation output double size=[3 1]; rhoInnovation output double size=1; innovationNorm output double size=1; traceP output double size=1; ekfPredictionValid output double size=1; ekfMeasurementUpdated output double size=1; ekfStateFinite output double size=1; minEigenvalueP output double size=1; symmetryErrorP output double size=1
function [ ...
    pHatW, ...
    vHatW, ...
    aHatW, ...
    pHatLeft, ...
    vHatLeft, ...
    rhoHatRaw, ...
    rhoHatSafe, ...
    innovation, ...
    rhoInnovation, ...
    innovationNorm, ...
    traceP, ...
    ekfPredictionValid, ...
    ekfMeasurementUpdated, ...
    ekfStateFinite, ...
    minEigenvalueP, ...
    symmetryErrorP] = fcn( ...
    zMeasured, ...
    measurementEnable, ...
    pWCL, ...
    RWCL, ...
    fMeasured, ...
    reset)
%#codegen
% V2九状态世界坐标系恒加速度EKF。
%
% 状态：
% x = [pW; vW; aW]
%
% 测量：
% zMeasured = [xLeft; yLeft; rhoStereo]
%
% fMeasured = [fxLeft; fxRight]，单位pixel。

%% 固定尺寸输出初始化
pHatW = zeros(3,1);
vHatW = zeros(3,1);
aHatW = zeros(3,1);

pHatLeft = zeros(3,1);
vHatLeft = zeros(3,1);

rhoHatRaw = 0;
rhoHatSafe = 0;

innovation = zeros(3,1);
rhoInnovation = 0;
innovationNorm = 0;

traceP = 0;

ekfPredictionValid = 0;
ekfMeasurementUpdated = 0;
ekfStateFinite = 0;

minEigenvalueP = 0;
symmetryErrorP = 0;

%% EKF持久状态
persistent x P

if isempty(x)
    x = cfg_ekfX0;
    P = cfg_ekfP0;
end

if reset > 0.5
    x = cfg_ekfX0;
    P = cfg_ekfP0;
end

%% 恒加速度状态模型
I3 = eye(3);
Z3 = zeros(3,3);
I9 = eye(9);

Ts = cfg_Ts;

F = [
    I3, Ts*I3, 0.5*Ts*Ts*I3
    Z3, I3,    Ts*I3
    Z3, Z3,    I3
];

sigmaJerkSquared = cfg_sigmaJerk * cfg_sigmaJerk;

Q = sigmaJerkSquared * [
    (Ts^5/20)*I3, (Ts^4/8)*I3, (Ts^3/6)*I3
    (Ts^4/8)*I3,  (Ts^3/3)*I3, (Ts^2/2)*I3
    (Ts^3/6)*I3,  (Ts^2/2)*I3, Ts*I3
];

%% 预测
xPred = F * x;
PPred = F * P * F' + Q;

% 强制保持协方差对称。
PPred = 0.5 * (PPred + PPred');

pPredW = xPred(1:3);

% 世界坐标目标位置转换到左相机坐标系。
pPredLeft = RWCL' * (pPredW - pWCL);

predictionFinite = ...
    all(isfinite(xPred)) && ...
    all(isfinite(PPred(:))) && ...
    all(isfinite(pPredLeft)) && ...
    all(isfinite(RWCL(:))) && ...
    all(isfinite(pWCL));

ekfPredictionValid = double( ...
    predictionFinite && ...
    pPredLeft(3) > cfg_visibilityZMin);

%% 构造测量模型
h = zeros(3,1);
H = zeros(3,9);

measurementOK = ...
    measurementEnable > 0.5 && ...
    ekfPredictionValid > 0.5 && ...
    all(isfinite(zMeasured)) && ...
    all(isfinite(fMeasured)) && ...
    all(fMeasured > cfg_numericalEpsilon);

if measurementOK
    Z = pPredLeft(3);
    rho = 1 / Z;

    xLeftPred = pPredLeft(1) / Z;
    yLeftPred = pPredLeft(2) / Z;

    h = [
        xLeftPred
        yLeftPred
        rho
    ];

    HLeft = [
        rho, 0,   -xLeftPred*rho
        0,   rho, -yLeftPred*rho
        0,   0,   -rho*rho
    ];

    HWorld = HLeft * RWCL';

    H = [
        HWorld, zeros(3,3), zeros(3,3)
    ];
end

%% 默认只采用预测结果
x = xPred;
P = PPred;

%% EKF测量更新
if measurementOK && ...
        all(isfinite(h)) && ...
        all(isfinite(H(:)))

    innovation = zMeasured - h;
    rhoInnovation = innovation(3);

    pixelVariance = ...
        cfg_pixelNoiseStd * cfg_pixelNoiseStd;

    fL = max( ...
        fMeasured(1), ...
        cfg_numericalEpsilon);

    fR = max( ...
        fMeasured(2), ...
        cfg_numericalEpsilon);

    baseline = max( ...
        cfg_baseline, ...
        cfg_numericalEpsilon);

    varXL = pixelVariance / (fL*fL);

    covXRho = ...
        pixelVariance / ...
        (baseline*fL*fL);

    varRho = ...
        pixelVariance / (baseline*baseline) * ...
        (1/(fL*fL) + 1/(fR*fR));

    R = [
        varXL,   0,        covXRho
        0,       varXL,    0
        covXRho, 0,        varRho
    ] + 1e-12 * eye(3);

    S = H * PPred * H' + R;

    if all(isfinite(S(:))) && ...
            rcond(S) > cfg_ekfSConditionMin

        K = (PPred * H') / S;

        x = xPred + K * innovation;

        % Joseph形式协方差更新。
        A = I9 - K * H;

        P = ...
            A * PPred * A' + ...
            K * R * K';

        P = 0.5 * (P + P');

        if cfg_ekfCovarianceJitter > 0
            P = P + ...
                cfg_ekfCovarianceJitter * I9;
        end

        ekfMeasurementUpdated = 1;
    end
end

%% 状态输出
pHatW = x(1:3);
vHatW = x(4:6);
aHatW = x(7:9);

pHatLeft = RWCL' * (pHatW - pWCL);
vHatLeft = RWCL' * vHatW;

ekfStateFinite = double( ...
    all(isfinite(x)) && ...
    all(isfinite(P(:))) && ...
    all(isfinite(pHatLeft)) && ...
    all(isfinite(vHatLeft)));

%% 逆深度输出
if ekfStateFinite > 0.5 && ...
        pHatLeft(3) > cfg_visibilityZMin

    rhoHatRaw = 1 / pHatLeft(3);

    rhoHatSafe = min( ...
        max(rhoHatRaw, cfg_rhoMin), ...
        cfg_rhoMax);
else
    rhoHatRaw = 0;
    rhoHatSafe = 0;
    ekfPredictionValid = 0;
end

%% EKF诊断
innovationNorm = ...
    sqrt(innovation' * innovation);

symmetryErrorP = ...
    norm(P - P', 'fro');

Psym = 0.5 * (P + P');

traceP = trace(Psym);

eigenvaluesP = eig(Psym);

minEigenvalueP = ...
    min(real(eigenvaluesP));

%% 非有限状态自动复位
if ekfStateFinite < 0.5
    x = cfg_ekfX0;
    P = cfg_ekfP0;

    pHatW = x(1:3);
    vHatW = x(4:6);
    aHatW = x(7:9);

    pHatLeft = zeros(3,1);
    vHatLeft = zeros(3,1);

    rhoHatRaw = 0;
    rhoHatSafe = 0;

    innovation = zeros(3,1);
    rhoInnovation = 0;
    innovationNorm = 0;

    symmetryErrorP = 0;
    traceP = trace(P);
    minEigenvalueP = 0;

    ekfPredictionValid = 0;
    ekfMeasurementUpdated = 0;
end
end

== matlab function stereo_ibvs_core_before_04_kinematics_20260723_212009/08_Zoom_Controller/08A Right Visibility Guard ==
  data: xLeftMeasured input; uRightPredicted output; rhoHatSafe input; focalLengthMeasuredMm input; validLeft input; validRight input; ekfPredictionValid input; rightReacquireActive input; resetSafe input; rightVisibilityMarginActualPx output; fRightMaxVisibleMm output; fRightMaxEffectiveMm output; rightScaleDesiredEffective output; rightVisibilityActive output; rightVisibilityInfeasible output; scaleDesiredEffective output; rightScaleDesiredNominal output; fRightMeasuredMm output
function [ ...
    uRightPredicted, ...
    rightVisibilityMarginActualPx, ...
    fRightMaxVisibleMm, ...
    fRightMaxEffectiveMm, ...
    rightScaleDesiredEffective, ...
    rightVisibilityActive, ...
    rightVisibilityInfeasible, ...
    scaleDesiredEffective, ...
    rightScaleDesiredNominal, ...
    fRightMeasuredMm] = fcn( ...
    xLeftMeasured, ...
    rhoHatSafe, ...
    focalLengthMeasuredMm, ...
    validLeft, ...
    validRight, ...
    ekfPredictionValid, ...
    rightReacquireActive, ...
    resetSafe)
%#codegen
% V2右相机可见性保护。

persistent active

if isempty(active)
    active = 1;
end

if resetSafe > 0.5
    active = 1;
end

rightScaleDesiredNominal = cfg_scaleDesired(2);
fRightMeasuredMm = focalLengthMeasuredMm(2);

rho = max(rhoHatSafe, cfg_numericalEpsilon);

% 校正平行双目的右相机归一化横坐标。
xRightPredicted = ...
    xLeftMeasured - cfg_baseline * rho;

fRightPx = ...
    focalLengthMeasuredMm(2) / ...
    cfg_outputPixelPitchXmm;

uRightPredicted = ...
    cfg_cxR + fRightPx * xRightPredicted;

rightVisibilityMarginActualPx = min( ...
    uRightPredicted, ...
    cfg_imageWidth - uRightPredicted);

hardwareMaxPx = ...
    cfg_focalLengthHardwareMaxMm(2) / ...
    cfg_outputPixelPitchXmm;

if xRightPredicted < -cfg_visibilityEpsilon

    fMaxPx = ...
        (cfg_cxR - cfg_rightVisibilityMarginPx) / ...
        (-xRightPredicted);

elseif xRightPredicted > cfg_visibilityEpsilon

    fMaxPx = ...
        (cfg_imageWidth - ...
        cfg_rightVisibilityMarginPx - ...
        cfg_cxR) / ...
        xRightPredicted;

else
    fMaxPx = hardwareMaxPx;
end

fMaxPx = max(fMaxPx, 0);

fRightMaxVisibleMm = ...
    fMaxPx * cfg_outputPixelPitchXmm;

rawEffective = min([
    cfg_focalLengthWorkingMaxMm(2)
    cfg_focalLengthHardwareMaxMm(2)
    fRightMaxVisibleMm
]);

rightVisibilityInfeasible = double( ...
    rawEffective < cfg_focalLengthWorkingMinMm(2));

fRightMaxEffectiveMm = max( ...
    cfg_focalLengthWorkingMinMm(2), ...
    rawEffective);

scaleRightMaxVisible = ...
    cfg_targetCharacteristicSize * ...
    fMaxPx * rho;

rightScaleDesiredEffective = min( ...
    rightScaleDesiredNominal, ...
    max(scaleRightMaxVisible, cfg_numericalEpsilon));

scaleDesiredEffective = [
    cfg_scaleDesired(1)
    rightScaleDesiredEffective
];

enterGuard = ...
    validLeft <= 0.5 || ...
    ekfPredictionValid <= 0.5 || ...
    validRight <= 0.5 || ...
    rightReacquireActive > 0.5 || ...
    rightVisibilityInfeasible > 0.5 || ...
    uRightPredicted < cfg_rightVisibilityMarginPx || ...
    uRightPredicted > ...
        cfg_imageWidth - cfg_rightVisibilityMarginPx || ...
    focalLengthMeasuredMm(2) > ...
        fRightMaxEffectiveMm + cfg_numericalEpsilon;

exitGuard = ...
    validLeft > 0.5 && ...
    validRight > 0.5 && ...
    ekfPredictionValid > 0.5 && ...
    rightReacquireActive <= 0.5 && ...
    rightVisibilityInfeasible <= 0.5 && ...
    uRightPredicted >= ...
        cfg_rightVisibilityMarginPx + ...
        cfg_rightVisibilityHysteresisPx && ...
    uRightPredicted <= ...
        cfg_imageWidth - ...
        cfg_rightVisibilityMarginPx - ...
        cfg_rightVisibilityHysteresisPx && ...
    focalLengthMeasuredMm(2) <= ...
        fRightMaxEffectiveMm;

if enterGuard
    active = 1;
elseif exitGuard
    active = 0;
end

rightVisibilityActive = double(active > 0.5);

if any(~isfinite([
        uRightPredicted
        rightVisibilityMarginActualPx
        fRightMaxVisibleMm
        fRightMaxEffectiveMm
        rightScaleDesiredEffective]))

    uRightPredicted = cfg_cxR;
    rightVisibilityMarginActualPx = 0;

    fRightMaxVisibleMm = 0;
    fRightMaxEffectiveMm = ...
        cfg_focalLengthWorkingMinMm(2);

    rightScaleDesiredEffective = ...
        cfg_numericalEpsilon;

    scaleDesiredEffective = [
        cfg_scaleDesired(1)
        rightScaleDesiredEffective
    ];

    rightVisibilityActive = 1;
    rightVisibilityInfeasible = 1;
end
end

== matlab function stereo_ibvs_core_before_04_kinematics_20260723_212009/10_Diagnostics/Stage1 Diagnostics ==
  data: inputDataValid input; controllerStatus output; cameraModelValid input; kinematicsValid input; validLeft input; validRight input; depthMeasurementValid input; centerTaskValid input; safetyValid input; ekfValid input; zoomControllerValid input; controllerEnable input; jConditionMetric input; systemReady output; faultCode output
function [controllerStatus,systemReady,faultCode] = ...
    fcn(inputDataValid,cameraModelValid,kinematicsValid, ...
    validLeft,validRight,depthMeasurementValid, ...
    centerTaskValid,safetyValid,ekfValid,zoomControllerValid, ...
    controllerEnable,jConditionMetric)
%#codegen
% 代码作用：
% 汇总Stage 1各子系统的有效状态，判断当前控制链路是否准备完成，
% 并输出统一的状态向量和故障代码，便于后续记录和ROS监控。

% 输入参数含义：
% inputDataValid：
% 顶层输入数据是否有效。
%
% cameraModelValid：
% 相机内参模型是否有效。
%
% kinematicsValid：
% FR3运动学和左相机雅可比是否有效。
%
% validLeft、validRight：
% 左右相机目标检测是否有效。
%
% depthMeasurementValid：
% 双目逆深度测量是否有效。
%
% centerTaskValid：
% 左相机中心任务计算是否有效。
%
% safetyValid：
% 安全模块是否允许输出关节速度。
%
% ekfValid：
% 目标运动EKF是否有效。
% Stage 1中固定为0。
%
% zoomControllerValid：
% 变焦控制器是否有效。
% Stage 1中固定为0。
%
% controllerEnable：
% 控制器总使能信号。
%
% jConditionMetric：
% 中心任务雅可比条件指标。

% 输出参数含义：
% controllerStatus：
% 统一状态向量，格式为：
% [inputDataValid;
%  cameraModelValid;
%  kinematicsValid;
%  validLeft;
%  validRight;
%  depthMeasurementValid;
%  centerTaskValid;
%  safetyValid;
%  ekfValid;
%  zoomControllerValid;
%  controllerEnable;
%  jConditionMetric]
%
% systemReady：
% Stage 1中心控制链路是否准备完成。
% 准备完成为1，否则为0。
%
% faultCode：
% 当前主要故障代码：
% 0：无故障
% 1：输入数据无效
% 2：相机模型无效
% 3：机械臂运动学无效
% 4：左相机目标无效
% 5：中心任务计算无效
% 6：安全模块未通过
% 7：控制器未使能

controllerStatus = zeros(12,1);
systemReady = 0;
faultCode = 0;

statusInputs = [
    inputDataValid
    cameraModelValid
    kinematicsValid
    validLeft
    validRight
    depthMeasurementValid
    centerTaskValid
    safetyValid
    ekfValid
    zoomControllerValid
    controllerEnable
    jConditionMetric
];

% 检查输入是否包含NaN或Inf。
if any(~isfinite(statusInputs))
    faultCode = 1;
    return;
end

controllerStatus = statusInputs;

% Stage 1只要求左相机中心控制链路有效。
systemReady = double( ...
    inputDataValid > 0.5 && ...
    cameraModelValid > 0.5 && ...
    kinematicsValid > 0.5 && ...
    validLeft > 0.5 && ...
    centerTaskValid > 0.5 && ...
    safetyValid > 0.5 && ...
    controllerEnable > 0.5);

% 按优先级输出主要故障原因。
if inputDataValid <= 0.5
    faultCode = 1;
elseif cameraModelValid <= 0.5
    faultCode = 2;
elseif kinematicsValid <= 0.5
    faultCode = 3;
elseif validLeft <= 0.5
    faultCode = 4;
elseif centerTaskValid <= 0.5
    faultCode = 5;
elseif safetyValid <= 0.5
    faultCode = 6;
elseif controllerEnable <= 0.5
    faultCode = 7;
else
    faultCode = 0;
end
end

== matlab function stereo_ibvs_core_before_04_kinematics_20260723_212009/08_Zoom_Controller/08B Zoom Controller ==
  data: focalLengthMeasuredMm input; scaleMeasured input; fDotMmCmd output; rhoHatSafe input; rhoDotHat input; scaleDesiredEffective input; validLeft input; ekfPredictionValid input; focalAtWorkingLowerLimit input; focalAtWorkingUpperLimit input; fRightMaxEffectiveMm input; rightVisibilityActive input; rightReacquireActive input; fDotMmLimited output; scaleError output; gDotCmd output; focalCommandOutwardAtWorkingLimit output; focalFeasible output; focalRateUsageGuaranteedCmd output; focalRateUsageHardCmd output
function [ ...
    fDotMmCmd, ...
    fDotMmLimited, ...
    scaleError, ...
    gDotCmd, ...
    focalCommandOutwardAtWorkingLimit, ...
    focalFeasible, ...
    focalRateUsageGuaranteedCmd, ...
    focalRateUsageHardCmd] = fcn( ...
    focalLengthMeasuredMm, ...
    scaleMeasured, ...
    rhoHatSafe, ...
    rhoDotHat, ...
    scaleDesiredEffective, ...
    validLeft, ...
    ekfPredictionValid, ...
    focalAtWorkingLowerLimit, ...
    focalAtWorkingUpperLimit, ...
    fRightMaxEffectiveMm, ...
    rightVisibilityActive, ...
    rightReacquireActive)
%#codegen
% V2独立对数焦距控制器。

fDotMmCmd = zeros(2,1);
fDotMmLimited = zeros(2,1);

scaleError = zeros(2,1);
gDotCmd = zeros(2,1);

focalCommandOutwardAtWorkingLimit = zeros(2,1);
focalFeasible = ones(2,1);

focalRateUsageGuaranteedCmd = zeros(2,1);
focalRateUsageHardCmd = zeros(2,1);

upperEffective = [
    cfg_focalLengthWorkingMaxMm(1)
    fRightMaxEffectiveMm
];

rho = max(rhoHatSafe, cfg_numericalEpsilon);

for cameraIndex = 1:2

    scaleCurrent = max( ...
        scaleMeasured(cameraIndex), ...
        cfg_numericalEpsilon);

    scaleDesired = max( ...
        scaleDesiredEffective(cameraIndex), ...
        cfg_numericalEpsilon);

    scaleError(cameraIndex) = ...
        log(scaleCurrent / scaleDesired);

    depthRateEstimate = ...
        rhoDotHat(cameraIndex) / rho;

    robustTerm = 0;

    if cfg_robustEnable > 0.5
        robustTerm = ...
            cfg_betaF(cameraIndex) * ...
            scaleError(cameraIndex) / ...
            (abs(scaleError(cameraIndex)) + ...
            cfg_epsilonF(cameraIndex));
    end

    gDotCmd(cameraIndex) = ...
        -cfg_Kf(cameraIndex,cameraIndex) * ...
        scaleError(cameraIndex) - ...
        depthRateEstimate - ...
        robustTerm;

    fDotMmCmd(cameraIndex) = ...
        focalLengthMeasuredMm(cameraIndex) * ...
        gDotCmd(cameraIndex);

    focalRequiredMm = ...
        scaleDesiredEffective(cameraIndex) / ...
        (cfg_targetCharacteristicSize * rho) * ...
        cfg_outputPixelPitchXmm;

    if focalRequiredMm < ...
            cfg_focalLengthWorkingMinMm(cameraIndex) || ...
            focalRequiredMm > upperEffective(cameraIndex)

        focalFeasible(cameraIndex) = 0;
    end

    focalCommandOutwardAtWorkingLimit(cameraIndex) = double( ...
        (focalAtWorkingLowerLimit(cameraIndex) > 0.5 && ...
        fDotMmCmd(cameraIndex) < 0) || ...
        (focalAtWorkingUpperLimit(cameraIndex) > 0.5 && ...
        fDotMmCmd(cameraIndex) > 0) || ...
        (focalLengthMeasuredMm(cameraIndex) >= ...
        upperEffective(cameraIndex) && ...
        fDotMmCmd(cameraIndex) > 0));
end

%% 右相机重捕获与可见性保护
if rightVisibilityActive > 0.5 || ...
        rightReacquireActive > 0.5

    if focalLengthMeasuredMm(2) > ...
            fRightMaxEffectiveMm + ...
            cfg_numericalEpsilon

        fDotMmCmd(2) = ...
            -cfg_rightReacquireZoomRateMmPerSec;
    else
        fDotMmCmd(2) = ...
            min(fDotMmCmd(2), 0);
    end
end

%% 左相机或EKF失效时，两相机安全缩焦
if validLeft <= 0.5 || ...
        ekfPredictionValid <= 0.5

    fDotMmCmd(1) = 0;

    if focalLengthMeasuredMm(1) > ...
            cfg_focalLengthWorkingMinMm(1)

        fDotMmCmd(1) = ...
            -cfg_rightReacquireZoomRateMmPerSec;
    end

    fDotMmCmd(2) = 0;

    if focalLengthMeasuredMm(2) > ...
            cfg_focalLengthWorkingMinMm(2)

        fDotMmCmd(2) = ...
            -cfg_rightReacquireZoomRateMmPerSec;
    end
end

%% 设计速度限制
fDotMmLimited = min( ...
    max( ...
        fDotMmCmd, ...
        -cfg_focalRateDesignMmPerSec), ...
    cfg_focalRateDesignMmPerSec);

% 防止下一采样周期越过右相机有效焦距上限。
nextRightFocalLength = ...
    focalLengthMeasuredMm(2) + ...
    cfg_Ts * fDotMmLimited(2);

if focalLengthMeasuredMm(2) <= ...
        fRightMaxEffectiveMm && ...
        nextRightFocalLength > ...
        fRightMaxEffectiveMm

    fDotMmLimited(2) = min( ...
        fDotMmLimited(2), ...
        (fRightMaxEffectiveMm - ...
        focalLengthMeasuredMm(2)) / cfg_Ts);
end

focalRateUsageGuaranteedCmd = ...
    abs(fDotMmLimited) / ...
    cfg_focalRateGuaranteedMmPerSec;

focalRateUsageHardCmd = ...
    abs(fDotMmLimited) / ...
    cfg_focalRateAbsoluteMaxMmPerSec;

%% 总开关与数值保护
if cfg_zoomControlEnable <= 0.5 || ...
        any(~isfinite(fDotMmCmd)) || ...
        any(~isfinite(fDotMmLimited))

    fDotMmCmd = zeros(2,1);
    fDotMmLimited = zeros(2,1);

    gDotCmd = zeros(2,1);

    focalRateUsageGuaranteedCmd = zeros(2,1);
    focalRateUsageHardCmd = zeros(2,1);
end
end
